simulink library "carnot"  (R2018b)
settings: Solver=VariableStepAuto  StartTime=0.0  StopTime=10.0  RelTol=1e-3
undefined symbols (not defined in the file or in its folder): A, A_earth, acol, Acol, ActPower1, ActPower2, ActPower3, Ad, Ad0, Ar, Au, Au0, Azimuth_Angle, B, Bd, Bd0, Br, Bu, Bu0, C, c1, c2, c3, c33, c4, c5, c6, CarnotCallbacks_Density, CarnotCallbacks_Enthalpy, CarnotCallbacks_Enthalpy2Temperature, CarnotCallbacks_Entropy, CarnotCallbacks_Evaporation_Enthalpy, CarnotCallbacks_GlobalMessageLevel, CarnotCallbacks_Grashof, CarnotCallbacks_Heat_Capacity, CarnotCallbacks_Kinematic_Viscosity, CarnotCallbacks_PMV_PPD, CarnotCallbacks_Prandtl, CarnotCallbacks_Saturation_Property, CarnotCallbacks_Saturation_Temperature, CarnotCallbacks_Saturation_Value_Water, CarnotCallbacks_Specific_Volume, CarnotCallbacks_Thermal_Conductivity, CarnotCallbacks_Vapour_Content, CarnotCallbacks_Vapour_Pressure, Cd, Cdl, Cr, Cu, Davies, Dd, DE_TRY2010_04_averageYear, delta_grd, density, DiameterLastPiece, dl, DPConstant, DPLinear, DPQuadratic, Dr ... (+59)
libraries: $bdroot x429, simulink x36, simulink_extras x12
(part 21 of 22)

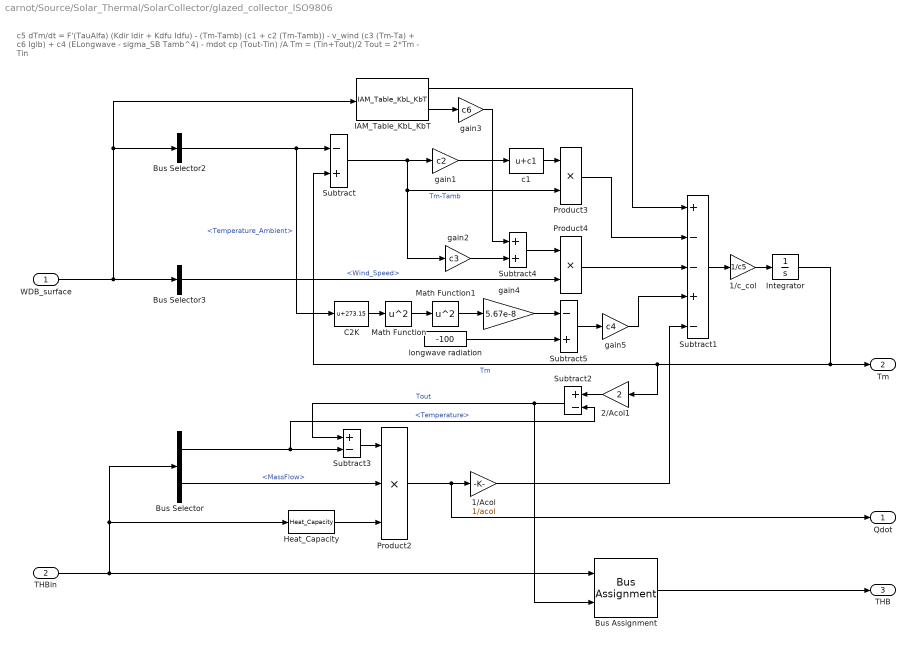
== system carnot/Source/Solar_Thermal/SolarCollector/glazed_collector_ISO9806 ==
  note: c5 dTm/dt = F'(TauAlfa) (Kdir Idir + Kdfu Idfu) - (Tm-Tamb) (c1 + c2 (Tm-Tamb)) - v_wind (c3 (Tm-Ta) + c6 Iglb) + c4 (ELongwave - sigma_SB Tamb^4) - mdot cp (Tout-Tin) /A
      | Tm = (Tin+Tout)/2
      | Tout = 2*Tm - Tin
  WDB_surface : Inport
  THBin : Inport  Port=2
  1/Acol : Gain  Gain=1/acol
  1/c_col : Gain  Gain=1/c5
  2/Acol1 : Gain  Gain=2
  Bus Assignment : BusAssignment  AssignedSignals=Temperature
  Bus Selector : BusSelector  OutputSignals=Temperature,MassFlow
  Bus Selector2 : BusSelector  OutputSignals=Temperature_Ambient
  Bus Selector3 : BusSelector  OutputSignals=Wind_Speed
  C2K : Bias  Bias=273.15
  Heat_Capacity : $bdroot/Basic/Material_Properties/Heat_Capacity  VariantControl=CarlibClassic  INPUTARGUMENTS=THB  DEBUGLEVEL=DEBUGLEVEL  MAXTOTALWARNINGS=inf  MAXCONSECUTIVEWARNINGS=inf  WRITETOFILE=0  FILENAME='errors.txt'
  IAM_Table_KbL_KbT : $bdroot/Source/Solar_Thermal/IncidenceAngleModifier/IAM_Table_KbL_KbT  fta=fta  kblangle=kblangle  KbL=KbL  kbtangle=kbtangle  KbT=KbT  Kd=Kd
  Integrator : Integrator  InitialCondition=tini
  Math Function : Math  Operator=square  SaturateOnIntegerOverflow=on
  Math Function1 : Math  Operator=square  SaturateOnIntegerOverflow=on
  Product2 : Product  Inputs=3  RndMeth=Zero
  Product3 : Product  RndMeth=Zero
  Product4 : Product  RndMeth=Zero
  Subtract : Sum  Inputs=-+
  Subtract1 : Sum  Inputs=+--+-
  Subtract2 : Sum  Inputs=+-
  Subtract3 : Sum  Inputs=+-
  Subtract4 : Sum  Inputs=2
  Subtract5 : Sum  Inputs=-+
  c1 : Bias  Bias=c1
  gain1 : Gain  Gain=c2
  gain2 : Gain  Gain=c3
  gain3 : Gain  Gain=c6
  gain4 : Gain  Gain=5.67e-8
  gain5 : Gain  Gain=c4
  longwave radiation : Constant  Value=-100
  Qdot : Outport  InitialOutput=0
  Tm : Outport  Port=2  InitialOutput=0
  THB : Outport  Port=3  InitialOutput=0
  wires:
  WDB_surface/1 -> Bus Selector3/1, IAM_Table_KbL_KbT/1, Bus Selector2/1
  Subtract4/1 -> Product4/1
  C2K/1 -> Math Function/1
  longwave radiation/1 -> Subtract5/2
  gain5/1 -> Subtract1/4
  Math Function/1 -> Math Function1/1
  2/Acol1/1 -> Subtract2/1
  Subtract/1 -> gain1/1, Product3/2, gain2/1  "Tm-Tamb"
  1/Acol/1 -> Subtract1/5
  Subtract2/1 -> Bus Assignment/2, Subtract3/1  "Tout"
  Heat_Capacity/1 -> Product2/3
  Integrator/1 -> Tm/1, 2/Acol1/1, Subtract/2  "Tm"
  Product2/1 -> Qdot/1, 1/Acol/1
  IAM_Table_KbL_KbT/2 -> gain3/1
  Subtract3/1 -> Product2/1
  Bus Selector2/1 -> C2K/1, Subtract/1  "<Temperature_Ambient>"
  gain1/1 -> c1/1
  gain2/1 -> Subtract4/2
  Product3/1 -> Subtract1/2
  1/c_col/1 -> Integrator/1
  Product4/1 -> Subtract1/3
  Math Function1/1 -> gain4/1
  THBin/1 -> Bus Assignment/1, Heat_Capacity/1, Bus Selector/1
  IAM_Table_KbL_KbT/1 -> Subtract1/1
  Bus Selector3/1 -> Product4/2  "<Wind_Speed>"
  Subtract5/1 -> gain5/1
  gain3/1 -> Subtract4/1
  gain4/1 -> Subtract5/1
  Subtract1/1 -> 1/c_col/1
  c1/1 -> Product3/1
  Bus Selector/1 -> Subtract2/2, Subtract3/2  "<Temperature>"
  Bus Selector/2 -> Product2/2  "<MassFlow>"
  Bus Assignment/1 -> THB/1

== system carnot/Source/Solar_Thermal/SolarCollector_2node/create_Cdat ==
  acol : Inport
  THBin : Inport  Port=2
  THBout : Inport  Port=3
  Qdot : Inport  Port=4
  Tmean : Inport  Port=5
  WDB : Inport  Port=6
  Bus Creator : BusCreator  Inputs=6
  Cdat : Outport
  wires:
  acol/1 -> Bus Creator/1  "Acol"
  THBin/1 -> Bus Creator/2  "THBin"
  THBout/1 -> Bus Creator/3  "THBout"
  WDB/1 -> Bus Creator/6  "WDB_surface"
  Bus Creator/1 -> Cdat/1
  Qdot/1 -> Bus Creator/4  "Qdot"
  Tmean/1 -> Bus Creator/5  "Tmean"

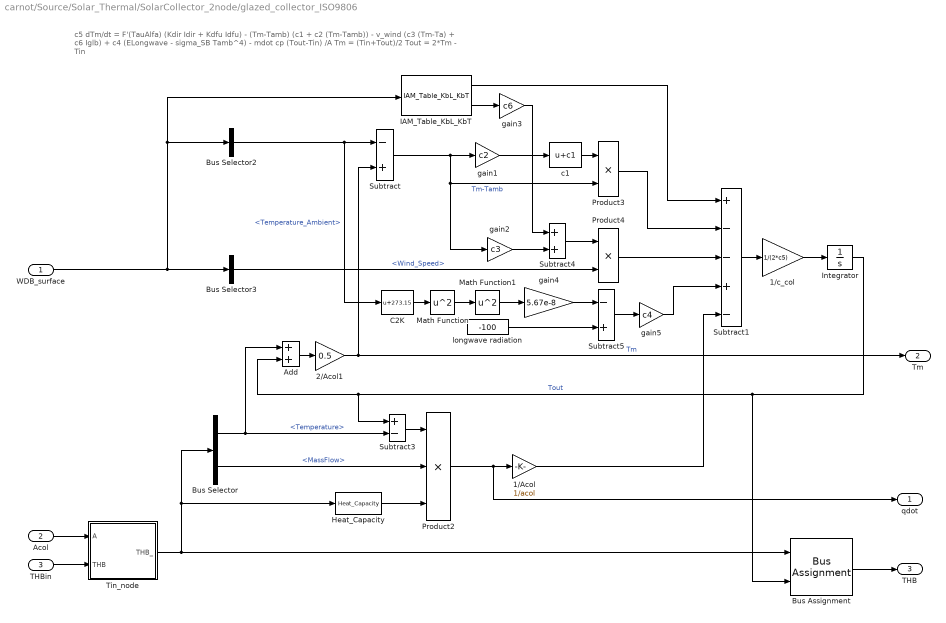
== system carnot/Source/Solar_Thermal/SolarCollector_2node/glazed_collector_ISO9806 ==
  note: c5 dTm/dt = F'(TauAlfa) (Kdir Idir + Kdfu Idfu) - (Tm-Tamb) (c1 + c2 (Tm-Tamb)) - v_wind (c3 (Tm-Ta) + c6 Iglb) + c4 (ELongwave - sigma_SB Tamb^4) - mdot cp (Tout-Tin) /A
      | Tm = (Tin+Tout)/2
      | Tout = 2*Tm - Tin
  WDB_surface : Inport
  Acol : Inport  Port=2
  THBin : Inport  Port=3
  1/Acol : Gain  Gain=1/acol
  1/c_col : Gain  Gain=1/(2*c5)
  2/Acol1 : Gain  Gain=0.5
  Add : Sum
  Bus Assignment : BusAssignment  AssignedSignals=Temperature
  Bus Selector : BusSelector  OutputSignals=Temperature,MassFlow
  Bus Selector2 : BusSelector  OutputSignals=Temperature_Ambient
  Bus Selector3 : BusSelector  OutputSignals=Wind_Speed
  C2K : Bias  Bias=273.15
  Heat_Capacity : $bdroot/Basic/Material_Properties/Heat_Capacity  VariantControl=CarlibClassic  INPUTARGUMENTS=THB  DEBUGLEVEL=DEBUGLEVEL  MAXTOTALWARNINGS=inf  MAXCONSECUTIVEWARNINGS=inf  WRITETOFILE=0  FILENAME='errors.txt'
  IAM_Table_KbL_KbT : $bdroot/Source/Solar_Thermal/IncidenceAngleModifier/IAM_Table_KbL_KbT  fta=fta  kblangle=kblangle  KbL=KbL  kbtangle=kbtangle  KbT=KbT  Kd=Kd
  Integrator : Integrator  InitialCondition=tini
  Math Function : Math  Operator=square  SaturateOnIntegerOverflow=on
  Math Function1 : Math  Operator=square  SaturateOnIntegerOverflow=on
  Product2 : Product  Inputs=3  RndMeth=Zero
  Product3 : Product  RndMeth=Zero
  Product4 : Product  RndMeth=Zero
  Subtract : Sum  Inputs=-+
  Subtract1 : Sum  Inputs=+--+-
  Subtract3 : Sum  Inputs=+-
  Subtract4 : Sum  Inputs=2
  Subtract5 : Sum  Inputs=-+
  Tin_node : Subsystem
  c1 : Bias  Bias=c1
  gain1 : Gain  Gain=c2
  gain2 : Gain  Gain=c3
  gain3 : Gain  Gain=c6
  gain4 : Gain  Gain=5.67e-8
  gain5 : Gain  Gain=c4
  longwave radiation : Constant  Value=-100
  qdot : Outport  InitialOutput=0
  Tm : Outport  Port=2  InitialOutput=0
  THB : Outport  Port=3  InitialOutput=0
  wires:
  Add/1 -> 2/Acol1/1
  2/Acol1/1 -> Subtract/2, Tm/1  "Tm"
  Acol/1 -> Tin_node/1(A)
  THBin/1 -> Tin_node/2(THB)
  WDB_surface/1 -> Bus Selector3/1, IAM_Table_KbL_KbT/1, Bus Selector2/1
  Subtract4/1 -> Product4/1
  C2K/1 -> Math Function/1
  longwave radiation/1 -> Subtract5/2
  gain5/1 -> Subtract1/4
  Math Function/1 -> Math Function1/1
  Subtract/1 -> gain1/1, Product3/2, gain2/1  "Tm-Tamb"
  1/Acol/1 -> Subtract1/5
  Heat_Capacity/1 -> Product2/3
  Integrator/1 -> Bus Assignment/2, Add/2, Subtract3/1  "Tout"
  Product2/1 -> qdot/1, 1/Acol/1
  IAM_Table_KbL_KbT/2 -> gain3/1
  Subtract3/1 -> Product2/1
  Bus Selector2/1 -> C2K/1, Subtract/1  "<Temperature_Ambient>"
  gain1/1 -> c1/1
  gain2/1 -> Subtract4/2
  Product3/1 -> Subtract1/2
  1/c_col/1 -> Integrator/1
  Product4/1 -> Subtract1/3
  Math Function1/1 -> gain4/1
  Tin_node/1(THB_) -> Heat_Capacity/1, Bus Selector/1, Bus Assignment/1
  IAM_Table_KbL_KbT/1 -> Subtract1/1
  Bus Selector3/1 -> Product4/2  "<Wind_Speed>"
  Subtract5/1 -> gain5/1
  gain3/1 -> Subtract4/1
  gain4/1 -> Subtract5/1
  Subtract1/1 -> 1/c_col/1
  c1/1 -> Product3/1
  Bus Selector/1 -> Add/1, Subtract3/2  "<Temperature>"
  Bus Selector/2 -> Product2/2  "<MassFlow>"
  Bus Assignment/1 -> THB/1

== system carnot/Source/Ventilation/Ventilation_AIV/Subsystem ==
  note: Remaining humidity or CO2 concentration
      | is difference of incomming x from outside (x_out)
      | and leaving x from inside (x_in)
  note: (kg/s)
  note: (kg/s)
  note: (kg/s)
  note: (kg/kg)
  note: (kg/kg)
  note: ASSUMPTION: mdot_air_out2in is equal to mdot_air_in2out
      | for the entire building
  mdot_air : Inport
  x_in : Inport  Port=2
  x_out : Inport  Port=3
  Constant : Constant  Value=0
  Demux2 : Demux  Outputs=2
  Demux3 : Demux  Outputs=2
  Product5 : Product  SaturateOnIntegerOverflow=on  InputSameDT=on  OutDataTypeStr=Inherit: Same as first input
  Product6 : Product  SaturateOnIntegerOverflow=on  InputSameDT=on  OutDataTypeStr=Inherit: Same as first input
  Sum1 : Sum  Inputs=+-  SaturateOnIntegerOverflow=on  InputSameDT=on  OutDataTypeStr=Inherit: Same as first input
  Sum2 : Sum  Inputs=+-  SaturateOnIntegerOverflow=on  InputSameDT=on  OutDataTypeStr=Inherit: Same as first input
  D_mdot_air : Outport
  D_mdot_H2O : Outport  Port=2
  D_mdot_CO2 : Outport  Port=3
  wires:
  x_out/1 -> Demux2/1
  Demux2/1 -> Sum1/1  "x_H2O_out"
  Demux2/2 -> Sum2/1  "x_CO2_out"
  Demux3/2 -> Sum2/2  "x_CO2_in"
  Demux3/1 -> Sum1/2  "x_H2O_in"
  x_in/1 -> Demux3/1
  Sum2/1 -> Product6/2
  Sum1/1 -> Product5/2
  mdot_air/1 -> Product5/1, Product6/1  "mdot_air"
  Product6/1 -> D_mdot_CO2/1  "mdot_CO2"
  Product5/1 -> D_mdot_H2O/1  "mdot_H2O"
  Constant/1 -> D_mdot_air/1

== system carnot/Storage/Thermal/Ice_Storage/Heat_Exchanger_HP ==
  note: 1.5 kW at 9 K on a 28 m tube
  Tice : Inport
  Tin : Inport  Port=2
  mdot : Inport  Port=3
  p : Inport  Port=4
  fluid : Inport  Port=5
  mix : Inport  Port=6
  Constant : Constant  Value=Lhx
  Constant1 : Constant  Value=mpc_hp
  Heat_Capacity : $bdroot/Basic/Material_Properties/Heat_Capacity  VariantControl=CarlibClassic  INPUTARGUMENTS=state variables (classic)  DEBUGLEVEL=DEBUGLEVEL  MAXTOTALWARNINGS=inf  MAXCONSECUTIVEWARNINGS=inf  WRITETOFILE=0  FILENAME='errors.txt'
  Integrator : Integrator  InitialCondition=t_ini
  Multiply : Product
  Multiply1 : Product  Inputs=/*/
  Product : Product  Inputs=3  SaturateOnIntegerOverflow=on  InputSameDT=on  OutDataTypeStr=Inherit: Same as first input
  Sum : Sum  Inputs=-+  SaturateOnIntegerOverflow=on  InputSameDT=on  OutDataTypeStr=Inherit: Same as first input
  Sum1 : Sum  Inputs=-+  SaturateOnIntegerOverflow=on  InputSameDT=on  OutDataTypeStr=Inherit: Same as first input
  Sum2 : Sum  Inputs=+-  SaturateOnIntegerOverflow=on  InputSameDT=on  OutDataTypeStr=Inherit: Same as first input
  U_length : Gain  Gain=Ulen  SaturateOnIntegerOverflow=on  OutDataTypeStr=Inherit: Same as input  ParamDataTypeStr=Inherit: Same as input
  Qdot2ice : Outport
  Thx : Outport  Port=2
  wires:
  Sum1/1 -> Multiply1/2
  Multiply1/1 -> Integrator/1
  Constant1/1 -> Multiply1/3
  Constant/1 -> Multiply/1, Multiply1/1
  Multiply/1 -> Sum1/1, Qdot2ice/1
  U_length/1 -> Multiply/2
  Tice/1 -> Sum2/2
  mix/1 -> Heat_Capacity/4
  fluid/1 -> Heat_Capacity/3
  p/1 -> Heat_Capacity/2
  mdot/1 -> Product/2
  Sum2/1 -> U_length/1
  Sum/1 -> Product/1
  Heat_Capacity/1 -> Product/3
  Product/1 -> Sum1/2
  Integrator/1 -> Thx/1, Sum2/1, Sum/1  "Thx"
  Tin/1 -> Sum/2, Heat_Capacity/1

== system carnot/Storage/Thermal/Ice_Storage/Heat_Exchanger_Solar ==
  note: 1.5 kW at 9 K on a 28 m tube
  Tice : Inport
  Tin : Inport  Port=2
  mdot : Inport  Port=3
  p : Inport  Port=4
  fluid : Inport  Port=5
  mix : Inport  Port=6
  Constant : Constant  Value=Lhx
  Constant1 : Constant  Value=mpc_hp
  Heat_Capacity : $bdroot/Basic/Material_Properties/Heat_Capacity  VariantControl=CarlibClassic  INPUTARGUMENTS=state variables (classic)  DEBUGLEVEL=DEBUGLEVEL  MAXTOTALWARNINGS=inf  MAXCONSECUTIVEWARNINGS=inf  WRITETOFILE=0  FILENAME='errors.txt'
  Integrator : Integrator  InitialCondition=t_ini
  Multiply : Product
  Multiply1 : Product  Inputs=/*/
  Product : Product  Inputs=3  SaturateOnIntegerOverflow=on  InputSameDT=on  OutDataTypeStr=Inherit: Same as first input
  Sum : Sum  Inputs=-+  SaturateOnIntegerOverflow=on  InputSameDT=on  OutDataTypeStr=Inherit: Same as first input
  Sum1 : Sum  Inputs=-+  SaturateOnIntegerOverflow=on  InputSameDT=on  OutDataTypeStr=Inherit: Same as first input
  Sum2 : Sum  Inputs=+-  SaturateOnIntegerOverflow=on  InputSameDT=on  OutDataTypeStr=Inherit: Same as first input
  U_length : Gain  Gain=Ulen  SaturateOnIntegerOverflow=on  OutDataTypeStr=Inherit: Same as input  ParamDataTypeStr=Inherit: Same as input
  Qdot2ice : Outport
  Thx : Outport  Port=2
  wires:
  Tin/1 -> Heat_Capacity/1, Sum/2
  Integrator/1 -> Sum/1, Sum2/1, Thx/1  "Thx"
  Product/1 -> Sum1/2
  Heat_Capacity/1 -> Product/3
  Sum/1 -> Product/1
  Sum2/1 -> U_length/1
  mdot/1 -> Product/2
  p/1 -> Heat_Capacity/2
  fluid/1 -> Heat_Capacity/3
  mix/1 -> Heat_Capacity/4
  Tice/1 -> Sum2/2
  U_length/1 -> Multiply/2
  Multiply/1 -> Qdot2ice/1, Sum1/1
  Constant/1 -> Multiply1/1, Multiply/1
  Constant1/1 -> Multiply1/3
  Multiply1/1 -> Integrator/1
  Sum1/1 -> Multiply1/2

== system carnot/Storage/Thermal/Ice_Storage/T_ground_undisturbed ==
  Fcn : Fcn  Expr=u(1) - u(2)*exp(-u(3)/u(4))*cos(2*pi*(u(5)-u(6)*3600)/(365*24*3600) - u(3)/u(4)) + 0.03*u(3)
  Mux : Mux  Inputs=6
  Tmeanoutside : Constant  Value=Tmeanoutside
  delta_grd : Constant  Value=delta_grd
  deltathetae : Constant  Value=deltathetae
  depth of center of wall : Constant  Value=ztilde
  time : Clock
  tshift : Constant  Value=tshift
  Tearth : Outport
  wires:
  Tmeanoutside/1 -> Mux/1
  deltathetae/1 -> Mux/2
  depth of center of wall/1 -> Mux/3
  delta_grd/1 -> Mux/4
  time/1 -> Mux/5
  tshift/1 -> Mux/6
  Mux/1 -> Fcn/1
  Fcn/1 -> Tearth/1

== system carnot/Storage/Thermal/Storage_Ports/Electric_Heating ==
  electric power : Inport
  THB : Inport  Port=2
  Bus Selector : BusSelector  OutputSignals=FluidType,FluidMix
  Gain : Gain  Gain=Q
  Mux3 : Mux  Inputs=8
  T_in : Constant  Value=ones(nodes,1)*20
  const2 : Constant  Value=1e5
  mdot : Constant  Value=zeros(nodes,1)
  to_storeT : Outport
  wires:
  Gain/1 -> Mux3/5  "Qdot_in"
  Bus Selector/2 -> Mux3/8  "<FluidMix>"
  electric power/1 -> Gain/1
  T_in/1 -> Mux3/1  "T_in"
  Mux3/1 -> to_storeT/1
  mdot/1 -> Mux3/4, Mux3/3, Mux3/2  "mdot_in"
  const2/1 -> Mux3/6
  THB/1 -> Bus Selector/1
  Bus Selector/1 -> Mux3/7  "<FluidType>"

== system carnot/Storage/Thermal/Storage_Ports/HX_EN12977 ==
  from_storeT : Inport
  THBin : Inport  Port=2
  Bus Assignment1 : BusAssignment  AssignedSignals=Temperature
  Mux3 : Mux  Inputs=8
  Pressure_Drop_StorageHX : $bdroot/Basic/Pressure_Drop/Pressure_Drop_StorageHX  dia=dia  hgt=height  dplin=dplin  dpqua=dpqua
  T_in : Constant  Value=zeros(nodes,1)
  fluid : Constant  Value=-9999
  mdot_in : Constant  Value=zeros(nodes,1)
  mix : Constant  Value=-9999
  p : Constant  Value=-9999
  select_Tout : Selector  InputPortWidth=nodes  IndexOptions=Index vector (dialog)  Indices=[outlet]  OutputSizes=1
  sfun_storage_heatexchanger : $bdroot/Basic/Thermal_Models/sfun_storage_heatexchanger  idn=heat transfer data fit EN12977  nodes=nodes  inlet=inlet  outlet=outlet  p1=ua0  p2=uam  p3=uat  p4=uat2  p5=0  p6=0  p7=0
  to_storeT : Outport
  THBout : Outport  Port=2
  wires:
  from_storeT/1 -> sfun_storage_heatexchanger/1
  THBin/1 -> Pressure_Drop_StorageHX/1, sfun_storage_heatexchanger/2
  mdot_in/1 -> Mux3/2, Mux3/3, Mux3/4  "mdot_in"
  Mux3/1 -> to_storeT/1
  select_Tout/1 -> Bus Assignment1/2
  T_in/1 -> Mux3/1  "T_in"
  sfun_storage_heatexchanger/1 -> Mux3/5  "Q_in"
  Bus Assignment1/1 -> THBout/1
  p/1 -> Mux3/6
  fluid/1 -> Mux3/7
  mix/1 -> Mux3/8
  sfun_storage_heatexchanger/2 -> select_Tout/1
  Pressure_Drop_StorageHX/1 -> Bus Assignment1/1

== system carnot/Storage/Thermal/Storage_Ports/HX_EN12977_stratified ==
  from_storeT : Inport
  THBin : Inport  Port=2
  Bus Assignment1 : BusAssignment  AssignedSignals=Temperature
  Mux3 : Mux  Inputs=8
  Pressure_Drop_StorageHX : $bdroot/Basic/Pressure_Drop/Pressure_Drop_StorageHX  dia=dia  hgt=height  dplin=dplin  dpqua=dpqua
  T_in : Constant  Value=zeros(nodes,1)
  fluid : Constant  Value=-9999
  mdot_in : Constant  Value=zeros(nodes,1)
  mix : Constant  Value=-9999
  p : Constant  Value=-9999
  select_Tout : Selector  InputPortWidth=nodes  IndexOptions=Index vector (dialog)  Indices=[outlet]  OutputSizes=1
  sfun_storage_heatexchanger : $bdroot/Basic/Thermal_Models/sfun_storage_heatexchanger  idn="heat transfer data fit EN12977  - stratified"  nodes=nodes  inlet=inlet  outlet=outlet  p1=ua0  p2=uam  p3=uat  p4=uat2  p5=0  p6=0  p7=0
  to_storeT : Outport
  THBout : Outport  Port=2
  wires:
  from_storeT/1 -> sfun_storage_heatexchanger/1
  THBin/1 -> Pressure_Drop_StorageHX/1, sfun_storage_heatexchanger/2
  mdot_in/1 -> Mux3/2, Mux3/3, Mux3/4  "mdot_in"
  Mux3/1 -> to_storeT/1
  select_Tout/1 -> Bus Assignment1/2
  T_in/1 -> Mux3/1  "T_in"
  sfun_storage_heatexchanger/1 -> Mux3/5  "Q_in"
  Bus Assignment1/1 -> THBout/1
  p/1 -> Mux3/6
  fluid/1 -> Mux3/7
  mix/1 -> Mux3/8
  sfun_storage_heatexchanger/2 -> select_Tout/1
  Pressure_Drop_StorageHX/1 -> Bus Assignment1/1

== system carnot/Storage/Thermal/Storage_Ports/HX_data_fit ==
  note: UA = uac + mdot*uam + (Thx-Tstorage)*uat
      | Qdot = UA * (Tstore-Thx)
  from_storeT : Inport
  THBin : Inport  Port=2
  Bus Assignment1 : BusAssignment  AssignedSignals=Temperature
  Mux3 : Mux  Inputs=8
  Pressure_Drop_StorageHX : $bdroot/Basic/Pressure_Drop/Pressure_Drop_StorageHX  dia=dia  hgt=height  dplin=dplin  dpqua=dpqua
  T_in : Constant  Value=zeros(nodes,1)
  fluid : Constant  Value=-9999
  mdot_in : Constant  Value=zeros(nodes,1)
  mix : Constant  Value=-9999
  p : Constant  Value=-9999
  select_Tout : Selector  InputPortWidth=nodes  IndexOptions=Index vector (dialog)  Indices=[outlet]  OutputSizes=1
  sfun_storage_heatexchanger : $bdroot/Basic/Thermal_Models/sfun_storage_heatexchanger  idn=heat transfer from data fit  nodes=nodes  inlet=inlet  outlet=outlet  p1=ua0  p2=uam  p3=uat  p4=0  p5=0  p6=0  p7=0
  to_storeT : Outport
  THBout : Outport  Port=2
  wires:
  sfun_storage_heatexchanger/2 -> select_Tout/1
  mix/1 -> Mux3/8
  fluid/1 -> Mux3/7
  p/1 -> Mux3/6
  Bus Assignment1/1 -> THBout/1
  sfun_storage_heatexchanger/1 -> Mux3/5  "Q_in"
  T_in/1 -> Mux3/1  "T_in"
  select_Tout/1 -> Bus Assignment1/2
  Mux3/1 -> to_storeT/1
  mdot_in/1 -> Mux3/4, Mux3/3, Mux3/2  "mdot_in"
  THBin/1 -> Pressure_Drop_StorageHX/1, sfun_storage_heatexchanger/2
  from_storeT/1 -> sfun_storage_heatexchanger/1
  Pressure_Drop_StorageHX/1 -> Bus Assignment1/1

== system carnot/Storage/Thermal/Storage_Ports/HX_data_fit_stratified ==
  note: statified charging !
      | heat transfer:
      | UA = uac + mdot*uam + (Thx-Tstorage)*uat
      | Qdot = UA * (Tstore-Thx)
  from_storeT : Inport
  THBin : Inport  Port=2
  Bus Assignment1 : BusAssignment  AssignedSignals=Temperature
  Mux3 : Mux  Inputs=8
  Pressure_Drop_StorageHX : $bdroot/Basic/Pressure_Drop/Pressure_Drop_StorageHX  dia=dia  hgt=height  dplin=dplin  dpqua=dpqua
  T_in : Constant  Value=zeros(nodes,1)
  fluid : Constant  Value=-9999
  mdot_in : Constant  Value=zeros(nodes,1)
  mix : Constant  Value=-9999
  p : Constant  Value=-9999
  select_Tout : Selector  InputPortWidth=nodes  IndexOptions=Index vector (dialog)  Indices=[outlet]  OutputSizes=1
  sfun_storage_heatexchanger : $bdroot/Basic/Thermal_Models/sfun_storage_heatexchanger  idn="heat transfer from data fit  - stratified"  nodes=nodes  inlet=inlet  outlet=outlet  p1=ua0  p2=uam  p3=uat  p4=0  p5=0  p6=0  p7=0
  to_storeT : Outport
  THBout : Outport  Port=2
  wires:
  from_storeT/1 -> sfun_storage_heatexchanger/1
  THBin/1 -> Pressure_Drop_StorageHX/1, sfun_storage_heatexchanger/2
  mdot_in/1 -> Mux3/2, Mux3/3, Mux3/4  "mdot_in"
  Mux3/1 -> to_storeT/1
  select_Tout/1 -> Bus Assignment1/2
  T_in/1 -> Mux3/1  "T_in"
  sfun_storage_heatexchanger/1 -> Mux3/5  "Q_in"
  p/1 -> Mux3/6
  fluid/1 -> Mux3/7
  mix/1 -> Mux3/8
  sfun_storage_heatexchanger/2 -> select_Tout/1
  Pressure_Drop_StorageHX/1 -> Bus Assignment1/1
  Bus Assignment1/1 -> THBout/1

== system carnot/Storage/Thermal/Storage_Ports/HX_finned_tube ==
  from_storeT : Inport
  THBin : Inport  Port=2
  Bus Assignment1 : BusAssignment  AssignedSignals=Temperature
  Mux3 : Mux  Inputs=8
  Pressure_Drop_StorageHX : $bdroot/Basic/Pressure_Drop/Pressure_Drop_StorageHX  dia=dpipe  hgt=height  dplin=dplin  dpqua=dpqua
  T_in : Constant  Value=zeros(nodes,1)
  fluid : Constant  Value=-9999
  mdot_in : Constant  Value=zeros(nodes,1)
  mix : Constant  Value=-9999
  p : Constant  Value=-9999
  select_Tout : Selector  InputPortWidth=nodes  IndexOptions=Index vector (dialog)  Indices=[outlet]  OutputSizes=1
  sfun_storage_heatexchanger : $bdroot/Basic/Thermal_Models/sfun_storage_heatexchanger  idn=finned tube theoretical  nodes=nodes  inlet=inlet  outlet=outlet  p1=dpipe  p2=swall  p3=lpipe  p4=cond  p5=dfin  p6=sfin  p7=nfin
  to_storeT : Outport
  THBout : Outport  Port=2
  wires:
  from_storeT/1 -> sfun_storage_heatexchanger/1
  THBin/1 -> Pressure_Drop_StorageHX/1, sfun_storage_heatexchanger/2
  mdot_in/1 -> Mux3/2, Mux3/3, Mux3/4  "mdot_in"
  Mux3/1 -> to_storeT/1
  select_Tout/1 -> Bus Assignment1/2
  T_in/1 -> Mux3/1  "T_in"
  sfun_storage_heatexchanger/1 -> Mux3/5  "Q_in"
  Bus Assignment1/1 -> THBout/1
  p/1 -> Mux3/6
  fluid/1 -> Mux3/7
  mix/1 -> Mux3/8
  sfun_storage_heatexchanger/2 -> select_Tout/1
  Pressure_Drop_StorageHX/1 -> Bus Assignment1/1

== system carnot/Storage/Thermal/Storage_Ports/HX_finned_tube_stratified ==
  from_storeT : Inport
  THBin : Inport  Port=2
  Bus Assignment1 : BusAssignment  AssignedSignals=Temperature
  Mux3 : Mux  Inputs=8
  Pressure_Drop_StorageHX : $bdroot/Basic/Pressure_Drop/Pressure_Drop_StorageHX  dia=dpipe  hgt=height  dplin=dplin  dpqua=dpqua
  T_in : Constant  Value=zeros(nodes,1)
  fluid : Constant  Value=-9999
  mdot_in : Constant  Value=zeros(nodes,1)
  mix : Constant  Value=-9999
  p : Constant  Value=-9999
  select_Tout : Selector  InputPortWidth=nodes  IndexOptions=Index vector (dialog)  Indices=[outlet]  OutputSizes=1
  sfun_storage_heatexchanger : $bdroot/Basic/Thermal_Models/sfun_storage_heatexchanger  idn="finned tube theoretical  - stratified"  nodes=nodes  inlet=inlet  outlet=outlet  p1=dpipe  p2=swall  p3=lpipe  p4=cond  p5=dfin  p6=sfin  p7=nfin
  to_storeT : Outport
  THBout : Outport  Port=2
  wires:
  Pressure_Drop_StorageHX/1 -> Bus Assignment1/1
  sfun_storage_heatexchanger/2 -> select_Tout/1
  mix/1 -> Mux3/8
  fluid/1 -> Mux3/7
  p/1 -> Mux3/6
  Bus Assignment1/1 -> THBout/1
  sfun_storage_heatexchanger/1 -> Mux3/5  "Q_in"
  T_in/1 -> Mux3/1  "T_in"
  select_Tout/1 -> Bus Assignment1/2
  Mux3/1 -> to_storeT/1
  mdot_in/1 -> Mux3/4, Mux3/3, Mux3/2  "mdot_in"
  THBin/1 -> sfun_storage_heatexchanger/2, Pressure_Drop_StorageHX/1
  from_storeT/1 -> sfun_storage_heatexchanger/1

== system carnot/Storage/Thermal/Storage_Ports/HX_tube ==
  from_storeT : Inport
  THBin : Inport  Port=2
  Bus Assignment1 : BusAssignment  AssignedSignals=Temperature
  Mux3 : Mux  Inputs=8
  Pressure_Drop_StorageHX : $bdroot/Basic/Pressure_Drop/Pressure_Drop_StorageHX  dia=dia  hgt=height  dplin=dplin  dpqua=dpqua
  T_in : Constant  Value=zeros(nodes,1)
  fluid : Constant  Value=-9999
  mdot_in : Constant  Value=zeros(nodes,1)
  mix : Constant  Value=-9999
  p : Constant  Value=-9999
  select_Tout : Selector  InputPortWidth=nodes  IndexOptions=Index vector (dialog)  Indices=[outlet]  OutputSizes=1
  sfun_storage_heatexchanger : $bdroot/Basic/Thermal_Models/sfun_storage_heatexchanger  idn=smooth tube theoretical  nodes=nodes  inlet=inlet  outlet=outlet  p1=dpipe  p2=swall  p3=lpipe  p4=cond  p5=0  p6=0  p7=0
  to_storeT : Outport
  THBout : Outport  Port=2
  wires:
  Pressure_Drop_StorageHX/1 -> Bus Assignment1/1
  sfun_storage_heatexchanger/2 -> select_Tout/1
  mix/1 -> Mux3/8
  fluid/1 -> Mux3/7
  p/1 -> Mux3/6
  Bus Assignment1/1 -> THBout/1
  sfun_storage_heatexchanger/1 -> Mux3/5  "Q_in"
  T_in/1 -> Mux3/1  "T_in"
  select_Tout/1 -> Bus Assignment1/2
  Mux3/1 -> to_storeT/1
  mdot_in/1 -> Mux3/4, Mux3/3, Mux3/2  "mdot_in"
  THBin/1 -> Pressure_Drop_StorageHX/1, sfun_storage_heatexchanger/2
  from_storeT/1 -> sfun_storage_heatexchanger/1

== system carnot/Storage/Thermal/Storage_Ports/HX_tube_stratified ==
  from_storeT : Inport
  THBin : Inport  Port=2
  Bus Assignment1 : BusAssignment  AssignedSignals=Temperature
  Mux3 : Mux  Inputs=8
  Pressure_Drop_StorageHX : $bdroot/Basic/Pressure_Drop/Pressure_Drop_StorageHX  dia=dia  hgt=height  dplin=dplin  dpqua=dpqua
  T_in : Constant  Value=zeros(nodes,1)
  fluid : Constant  Value=-9999
  mdot_in : Constant  Value=zeros(nodes,1)
  mix : Constant  Value=-9999
  p : Constant  Value=-9999
  select_Tout : Selector  InputPortWidth=nodes  IndexOptions=Index vector (dialog)  Indices=[outlet]  OutputSizes=1
  sfun_storage_heatexchanger : $bdroot/Basic/Thermal_Models/sfun_storage_heatexchanger  idn=smooth tube theoretical - stratified  nodes=nodes  inlet=inlet  outlet=outlet  p1=dpipe  p2=swall  p3=lpipe  p4=cond  p5=0  p6=0  p7=0
  to_storeT : Outport
  THBout : Outport  Port=2
  wires:
  from_storeT/1 -> sfun_storage_heatexchanger/1
  THBin/1 -> sfun_storage_heatexchanger/2, Pressure_Drop_StorageHX/1
  mdot_in/1 -> Mux3/2, Mux3/3, Mux3/4  "mdot_in"
  Mux3/1 -> to_storeT/1
  select_Tout/1 -> Bus Assignment1/2
  T_in/1 -> Mux3/1  "T_in"
  sfun_storage_heatexchanger/1 -> Mux3/5  "Q_in"
  Bus Assignment1/1 -> THBout/1
  p/1 -> Mux3/6
  fluid/1 -> Mux3/7
  mix/1 -> Mux3/8
  sfun_storage_heatexchanger/2 -> select_Tout/1
  Pressure_Drop_StorageHX/1 -> Bus Assignment1/1

== system carnot/Storage/Thermal/Storage_Ports/Pipe_Connection ==
  from_storeT : Inport
  THBin : Inport  Port=2
  Bus Assignment : BusAssignment  AssignedSignals=Temperature
  Bus Selector : BusSelector  OutputSignals=Temperature,MassFlow,Pressure,FluidType,FluidMix
  Gain : Gain  Gain=in
  Gain1 : Gain  Gain=up
  Gain2 : Gain  Gain=down
  Gain3 : Gain  Gain=in
  Mux3 : Mux  Inputs=8
  Pressure_Drop_StoragePipe : $bdroot/Basic/Pressure_Drop/Pressure_Drop_StoragePipe  dpipe=dpipe  dstg=dstg  hgt=height
  Q_in : Constant  Value=zeros(nodes,1)
  select_Tin_2_Tout : Selector  InputPortWidth=nodes  IndexOptions=Index vector (dialog)  Indices=[idx_in_out]  OutputSizes=1
  select_Tout : Selector  InputPortWidth=nodes  IndexOptions=Index vector (dialog)  Indices=[outlet]  OutputSizes=1
  to_storeT : Outport
  THBout : Outport  Port=2
  wires:
  select_Tin_2_Tout/1 -> Pressure_Drop_StoragePipe/1
  Bus Selector/5 -> Mux3/8  "<FluidMix>"
  Bus Assignment/1 -> THBout/1
  Q_in/1 -> Mux3/5
  Gain3/1 -> Mux3/1  "T_in"
  select_Tout/1 -> Bus Assignment/2
  Mux3/1 -> to_storeT/1
  Gain2/1 -> Mux3/4  "mdot_down"
  Gain1/1 -> Mux3/3  "mdot_up"
  Gain/1 -> Mux3/2  "mdot_in"
  Bus Selector/1 -> Gain3/1  "<Temperature>"
  Bus Selector/2 -> Gain2/1, Gain1/1, Gain/1  "<MassFlow>"
  Bus Selector/3 -> Mux3/6  "<Pressure>"
  Bus Selector/4 -> Mux3/7  "<FluidType>"
  THBin/1 -> Bus Selector/1, Pressure_Drop_StoragePipe/2
  from_storeT/1 -> select_Tin_2_Tout/1, select_Tout/1
  Pressure_Drop_StoragePipe/1 -> Bus Assignment/1

== system carnot/Storage/Thermal/Storage_Ports/Pipe_stratified ==
  note: _________________________________
      | mdot_in ->                                                .
      | node 5                     .
      | __ mdot_down(4) V  ___mdot_up(4) ^ __
      | V                           ^    .
      | node 4                    .
      | __ mdot_down(3) V  ___mdot_up(3) ^ __
      | V                           ^    .
      | node 3                    .
      | __ mdot_down(2) V  ___mdot_up(2) ^ __
      | V                           ^    .
      | node 2                    .
      | __ mdot_down(1) V  ___mdot_up(1) ^ __
      | V                           ^    .
      | node 1                    .
      | _________________________________
  from_storeT : Inport
  THBin : Inport  Port=2
  Add : Sum  Inputs=-+
  Add2 : Sum  Inputs=1
  Bus Assignment : BusAssignment  AssignedSignals=Temperature
  Bus Selector : BusSelector  OutputSignals=Temperature,MassFlow,Pressure,FluidType,FluidMix
  Constant : Constant  Value=flowdir
  Gain1 : Gain  Gain=up
  Gain2 : Gain  Gain=flowdir
  Gain3 : Gain  Gain=ones(nodes,1)
  Gain5 : Gain  Gain=down
  If : If  NumInputs=2  IfExpression=u1 == 0  ElseIfExpressions=u2 < 0
  MinMax : MinMax  Function=max  Inputs=3
  Mux3 : Mux  Inputs=8
  Pressure_Drop_StoragePipe : $bdroot/Basic/Pressure_Drop/Pressure_Drop_StoragePipe  dpipe=dpipe  dstg=dstg  hgt=height
  Product : Product  RndMeth=Zero
  Product1 : Product  RndMeth=Zero
  Product2 : Product  RndMeth=Zero
  Q_in : Constant  Value=zeros(nodes,1)
  Relay : Relay  OnSwitchValue=0.05  OffSwitchValue=-0.05
  T_criteria not satisfied : Subsystem  TreatAsAtomicUnit=on
  index_to_internal_massflow : MATLABFcn  MATLABFcn=[u(2:end);0]  OutputDimensions=nodes
  massflow downwards : Subsystem  TreatAsAtomicUnit=on
  massflow upwards : Subsystem  TreatAsAtomicUnit=on
  select_Tin_2_Tout : Selector  InputPortWidth=nodes  IndexOptions=Index vector (dialog)  Indices=[idx_in_out]  OutputSizes=1
  select_Tn : Selector  InputPortWidth=nodes  IndexOptions=Index vector (dialog)  Indices=[1:nodes]  OutputSizes=1
  select_Tn_concerned : Selector  InputPortWidth=nodes  IndexOptions=Index vector (dialog)  Indices=n_concerned  OutputSizes=1
  select_Tout : Selector  InputPortWidth=nodes  IndexOptions=Index vector (dialog)  Indices=[outlet]  OutputSizes=1
  to_storeT : Outport
  THBout : Outport  Port=2
  wires:
  select_Tin_2_Tout/1 -> Pressure_Drop_StoragePipe/1
  Pressure_Drop_StoragePipe/1 -> Bus Assignment/1
  select_Tn_concerned/1 -> Add2/1, massflow downwards/1(In1), massflow upwards/1(In1)
  MinMax/1 -> Product1/2
  Add2/1 -> If/1
  Product1/1 -> Mux3/2  "mdot_in"
  Gain5/1 -> Product/2
  Relay/1 -> select_Tn_concerned/1, index_to_internal_massflow/1
  Product/1 -> Mux3/4  "mdot_down"
  from_storeT/1 -> select_Tin_2_Tout/1, select_Tn/1, select_Tout/1
  THBin/1 -> Pressure_Drop_StoragePipe/2, Bus Selector/1
  Bus Selector/4 -> Mux3/7  "<FluidType>"
  Bus Selector/3 -> Mux3/6  "<Pressure>"
  Bus Selector/2 -> Product/1, Product2/1, Product1/1  "<MassFlow>"
  Bus Selector/1 -> Gain3/1, Add/1  "<Temperature>"
  Mux3/1 -> to_storeT/1
  select_Tout/1 -> Bus Assignment/2
  Gain3/1 -> Mux3/1  "T_in"
  Q_in/1 -> Mux3/5
  Bus Assignment/1 -> THBout/1
  Bus Selector/5 -> Mux3/8  "<FluidMix>"
  select_Tn/1 -> Add/2
  Add/1 -> Gain2/1
  If/1 -> T_criteria not satisfied/Action
  Constant/1 -> If/2
  T_criteria not satisfied/1(Out1) -> MinMax/1
  If/2 -> massflow downwards/Action
  If/3 -> massflow upwards/Action
  massflow downwards/1(Out1) -> MinMax/2
  Gain1/1 -> Product2/2
  Product2/1 -> Mux3/3  "mdot_up"
  massflow upwards/1(Out1) -> MinMax/3
  Gain2/1 -> Relay/1
  index_to_internal_massflow/1 -> Gain5/1, Gain1/1

== system carnot/Storage/Thermal/Storage_Type_5/HX_EN12977_3 ==
  from_storeT : Inport
  THBin : Inport  Port=2
  Bus Assignment1 : BusAssignment  AssignedSignals=Temperature
  Mux3 : Mux  Inputs=8
  Pressure_Drop_StorageHX : $bdroot/Basic/Pressure_Drop/Pressure_Drop_StorageHX  dia=dia  hgt=height  dplin=dplin  dpqua=dpqua
  T_in : Constant  Value=zeros(nodes,1)
  fluid : Constant  Value=-9999
  mdot_in : Constant  Value=zeros(nodes,1)
  mix : Constant  Value=-9999
  p : Constant  Value=-9999
  select_Tout : Selector  InputPortWidth=nodes  IndexOptions=Index vector (dialog)  Indices=[outlet]  OutputSizes=1
  sfun_storage_heatexchanger : $bdroot/Basic/Thermal_Models/sfun_storage_heatexchanger  idn=heat transfer data fit EN12977  nodes=nodes  inlet=inlet  outlet=outlet  p1=ua0  p2=uam  p3=uat  p4=uat2  p5=0  p6=0  p7=0
  to_storeT : Outport
  THBout : Outport  Port=2
  wires:
  from_storeT/1 -> sfun_storage_heatexchanger/1
  THBin/1 -> Pressure_Drop_StorageHX/1, sfun_storage_heatexchanger/2
  mdot_in/1 -> Mux3/2, Mux3/3, Mux3/4  "mdot_in"
  Mux3/1 -> to_storeT/1
  select_Tout/1 -> Bus Assignment1/2
  T_in/1 -> Mux3/1  "T_in"
  sfun_storage_heatexchanger/1 -> Mux3/5  "Q_in"
  Bus Assignment1/1 -> THBout/1
  p/1 -> Mux3/6
  fluid/1 -> Mux3/7
  mix/1 -> Mux3/8
  sfun_storage_heatexchanger/2 -> select_Tout/1
  Pressure_Drop_StorageHX/1 -> Bus Assignment1/1

== system carnot/Storage/Thermal/detailed_storage_models/heat_exchanger_storage ==
  Tamb : Inport
  THBex_in : Inport  Port=2
  THBstg_in : Inport  Port=3
  Demux : Demux
  Demux1 : Demux  Outputs=[1 1 1 1 1 1]
  Demux2 : Demux  Outputs=[1 1 1 1 1 1]
  Demux3 : Demux  Outputs=[6 14]
  Demux4 : Demux  Outputs=[6 14]
  Mux1 : Mux  Inputs=7
  Mux2 : Mux  Inputs=7
  Mux3 : Mux  Inputs=13
  S-Function : S-Function  FunctionName=ministg  Parameters=v(1), v(2), loss, uh(1), uh(2), uc(1), uc(2), uw(1), uw(2), mat, m(1), m(2), t0, dph(1), dph(2), dph(3), dpc(1), dpc(2), dpc(3), n  SFunctionDeploymentMode=off  EnableBusSupport=off
  THB2THV : $bdroot/Toolbox/THB2THV
  THB2THV1 : $bdroot/Toolbox/THB2THV
  THV2THB : $bdroot/Toolbox/THV2THB
  THV2THB1 : $bdroot/Toolbox/THV2THB
  THBex : Outport
  THBstg : Outport  Port=2
  wires:
  Mux3/1 -> S-Function/1
  Demux2/6 -> Mux2/6, Mux3/13  "fluidmix"
  Demux1/6 -> Mux1/6, Mux3/7  "fluidmix"
  THV2THB1/1 -> THBstg/1
  THV2THB/1 -> THBex/1
  THB2THV1/1 -> Demux4/1
  THB2THV/1 -> Demux3/1
  Demux2/5 -> Mux2/5, Mux3/12  "fluidtype"
  Demux2/3 -> Mux2/3, Mux3/10  "mdot"
  Demux1/5 -> Mux1/5, Mux3/6  "fluidtype"
  Demux1/3 -> Mux1/3, Mux3/4  "mdot"
  Demux1/4 -> Mux3/5
  Demux1/2 -> Mux3/3
  Tamb/1 -> Mux3/1
  Demux1/1 -> Mux1/1, Mux3/2  "ID"
  Demux2/4 -> Mux3/11
  Demux2/2 -> Mux3/9
  Demux2/1 -> Mux2/1, Mux3/8  "ID"
  S-Function/1 -> Demux/1
  Demux3/1 -> Demux1/1
  THBex_in/1 -> THB2THV/1
  THBstg_in/1 -> THB2THV1/1
  Demux4/1 -> Demux2/1
  Demux/4 -> Mux2/4
  Demux/3 -> Mux2/2
  Mux2/1 -> THV2THB1/1
  Mux1/1 -> THV2THB/1
  Demux/2 -> Mux1/4
  Demux/1 -> Mux1/2
  Demux3/2 -> Mux1/7
  Demux4/2 -> Mux2/7

== system carnot/Storage/Thermal/surface_models/Isolated_Cover ==
  Tamb : Inport
  Mux2 : Mux  Inputs=2
  const1 : Constant  Value=[u 0]
  Tamb_utop_Iabs : Outport
  wires:
  Mux2/1 -> Tamb_utop_Iabs/1
  const1/1 -> Mux2/2
  Tamb/1 -> Mux2/1

== system carnot/Storage/Thermal/surface_models/Open_Surface ==
  WDB : Inport
  3*vwind : Gain  Gain=3  SaturateOnIntegerOverflow=on  OutDataTypeStr=Inherit: Same as input  ParamDataTypeStr=Inherit: Same as input
  Bus Selector : BusSelector  OutputSignals=Solar_Radiation_direct_surface,Solar_Radiation_diffuse_surface,Temperature_Ambient,Wind_Speed
  Fixed_Surface : $bdroot/Weather/Fixed_Surface  colangle=0  colazi=0  colrot=0
  Mux2 : Mux  Inputs=3
  Radiation_on_Inclined_Surface : $bdroot/Weather/Radiation_on_Inclined_Surface  sky=Perez 1990  reflect=0.2
  Sum : Sum  Inputs=2  SaturateOnIntegerOverflow=on  InputSameDT=on  OutDataTypeStr=Inherit: Same as first input
  add 5.6 : Subsystem  mask(add constant){c=5.6}
      mask prompts: c "constant c"
      mask help: This block adds a constant c to each element of the input vector.
      mask Help: file:///constant.htm
      mask Display: disp('+c');
  ground absorbtion : Gain  Gain=albedo  SaturateOnIntegerOverflow=on  OutDataTypeStr=Inherit: Same as input  ParamDataTypeStr=Inherit: Same as input
  Tamb_utop_Iabs : Outport
  wires:
  Bus Selector/2 -> Sum/2  "<Solar_Radiation_diffuse_surface>"
  WDB/1 -> Radiation_on_Inclined_Surface/1
  Fixed_Surface/1 -> Radiation_on_Inclined_Surface/2
  Radiation_on_Inclined_Surface/1 -> Bus Selector/1
  Bus Selector/3 -> Mux2/1  "<Temperature_Ambient>"
  ground absorbtion/1 -> Mux2/3
  Bus Selector/1 -> Sum/1  "<Solar_Radiation_direct_surface>"
  Sum/1 -> ground absorbtion/1
  3*vwind/1 -> add 5.6/1(In1)
  add 5.6/1(Out1) -> Mux2/2
  Mux2/1 -> Tamb_utop_Iabs/1
  Bus Selector/4 -> 3*vwind/1  "<Wind_Speed>"

== system carnot/Basic/Thermal_Models/Combustion_Calculation/exhaust gas/fluid//solid ==
  c : Inport
  h : Inport  Port=2
  s : Inport  Port=3
  n : Inport  Port=4
  w : Inport  Port=5
  Mux : Mux  Inputs=2
  Mux1 : Mux
  kgCO2 : Gain  Gain=3.67  SaturateOnIntegerOverflow=on  OutDataTypeStr=Inherit: Same as input  ParamDataTypeStr=Inherit: Same as input
  kgH2O : Fcn  Expr=9*u(1)+u(2)
  kgSO2 : Gain  Gain=2  SaturateOnIntegerOverflow=on  OutDataTypeStr=Inherit: Same as input  ParamDataTypeStr=Inherit: Same as input
  Out1 : Outport
  wires:
  n/1 -> Mux1/4
  s/1 -> kgSO2/1
  w/1 -> Mux/2
  Mux1/1 -> Out1/1
  h/1 -> Mux/1
  c/1 -> kgCO2/1
  kgSO2/1 -> Mux1/3
  kgH2O/1 -> Mux1/2
  kgCO2/1 -> Mux1/1
  Mux/1 -> kgH2O/1

== system carnot/Basic/Thermal_Models/Combustion_Calculation/exhaust gas/gas ==
  c : Inport
  h : Inport  Port=2
  s : Inport  Port=3
  n : Inport  Port=4
  Mux1 : Mux
  Terminator1 : Terminator
  kgCO2 : Gain  Gain=3.67  SaturateOnIntegerOverflow=on  OutDataTypeStr=Inherit: Same as input  ParamDataTypeStr=Inherit: Same as input
  kgH2O : Gain  Gain=9  SaturateOnIntegerOverflow=on  OutDataTypeStr=Inherit: Same as input  ParamDataTypeStr=Inherit: Same as input
  kgSO2 : Ground
  Out1 : Outport
  wires:
  n/1 -> Mux1/4
  kgSO2/1 -> Mux1/3
  kgH2O/1 -> Mux1/2
  kgCO2/1 -> Mux1/1
  Mux1/1 -> Out1/1
  s/1 -> Terminator1/1
  h/1 -> kgH2O/1
  c/1 -> kgCO2/1

== system carnot/Basic/Thermal_Models/HeatPump_basic/model cold side/add constant ==
  In1 : Inport
  Sum : Sum  SaturateOnIntegerOverflow=on  InputSameDT=on  OutDataTypeStr=Inherit: Same as first input
  const : Constant  Value=c
  Out1 : Outport
  wires:
  const/1 -> Sum/1
  In1/1 -> Sum/2
  Sum/1 -> Out1/1

== system carnot/Basic/Thermal_Models/Room_Node/convective_node/PressureCalculation ==
  D_mdot_air : Inport
  density : Inport  Port=2
  zoneairvolume : Inport  Port=3
  T : Inport  Port=4
  Enable : EnablePort
  Multiply : Product
  Subsystem : Subsystem
  m_air : Integrator  InitialConditionSource=external  InitialCondition=zonestartAIR  LimitOutput=on  LowerSaturationLimit=0
  x : Product  Inputs=*/*  SaturateOnIntegerOverflow=on  InputSameDT=on  OutDataTypeStr=Inherit: Same as first input
  p : Outport
  wires:
  D_mdot_air/1 -> m_air/1
  T/1 -> Subsystem/1(T)
  x/1 -> p/1
  density/1 -> Multiply/1
  m_air/1 -> x/1
  zoneairvolume/1 -> x/2, Multiply/2
  Multiply/1 -> m_air/2
  Subsystem/1(R*T ') -> x/3

== system carnot/Source/Chiller/Absorption_Chiller_LookUp/Lookup_table Q_hot + Q_cold + Recooling/NTDeadTime ==
  control_AC_runtime : Inport
  T_HT_IN : Inport  Port=2
  Compare To Constant : simulink/Logic and Bit Operations/Compare To Constant  relop=<  const=1  OutDataTypeStr=boolean
  Compare To Constant1 : simulink/Logic and Bit Operations/Compare To Constant  relop=>=  const=1  OutDataTypeStr=boolean
  Compare To Constant2 : simulink/Logic and Bit Operations/Compare To Constant  relop=>  const=eps(1)  OutDataTypeStr=boolean
  Constant : Constant  Value=data.deadtime_exponent
  Constant1 : Constant  Value=0.0
  Display{,1..3,5..6} (6 alike) : Display
  Gain_11768 : Gain  Gain=data.deadtime_factor
  Logical Operator : Logic  AllPortsSameDT=off  OutDataTypeStr=boolean
  Logical Operator1 : Logic  AllPortsSameDT=off  OutDataTypeStr=boolean
  Logical Operator2 : Logic  AllPortsSameDT=off  OutDataTypeStr=boolean
  Logical Operator3 : Logic  Operator=OR  AllPortsSameDT=off  OutDataTypeStr=boolean
  Math Function : Math  Operator=pow  SaturateOnIntegerOverflow=on
  Memory : Memory
  Memory1 : Memory
  Memory2 : Memory
  Relational Operator : RelationalOperator  OutDataTypeStr=boolean  RndMeth=Simplest
  Switch : Switch  Criteria=u2 > Threshold  Threshold=0.5
  Switch1 : Switch  Criteria=u2 > Threshold  Threshold=eps(1)
  Q_cold_on : Outport
  wires:
  T_HT_IN/1 -> Math Function/1
  Constant/1 -> Math Function/2
  Math Function/1 -> Gain_11768/1
  Gain_11768/1 -> Display/1, Switch/1
  Memory/1 -> Compare To Constant/1
  Compare To Constant/1 -> Logical Operator/1
  Logical Operator/1 -> Switch/2
  Switch/1 -> Switch1/1, Memory1/1, Display1/1
  Memory1/1 -> Switch/3
  control_AC_runtime/1 -> Display2/1, Compare To Constant2/1, Relational Operator/1, Switch1/2, Display5/1, Compare To Constant1/1, Memory/1
  Constant1/1 -> Switch1/3
  Compare To Constant1/1 -> Logical Operator/2
  Switch1/1 -> Display6/1, Relational Operator/2
  Relational Operator/1 -> Logical Operator1/2
  Compare To Constant2/1 -> Logical Operator1/1, Logical Operator2/2
  Memory2/1 -> Logical Operator2/1
  Logical Operator2/1 -> Logical Operator3/1
  Logical Operator3/1 -> Memory2/1, Display3/1, Q_cold_on/1
  Logical Operator1/1 -> Logical Operator3/2

== system carnot/Source/Chiller/Absorption_Chiller_LookUp/Lookup_table Q_hot + Q_cold + Recooling/runtime_AC ==
  control_AC : Inport
  Integrator : Integrator  ExternalReset=either
  runtime : Outport
  wires:
  control_AC/1 -> Integrator/2, Integrator/1
  Integrator/1 -> runtime/1

== system carnot/Source/Chiller/Absorption_Chiller_ddT/absorber // condenser/Tcooler_out ==
  T : Inport
  mdot : Inport  Port=2
  Qdot_E + Qdot_G : Inport  Port=3
  p : Inport  Port=4
  fluid : Inport  Port=5
  mix : Inport  Port=6
  Heat_Capacity : $bdroot/Basic/Material_Properties/Heat_Capacity  VariantControl=CarlibClassic  INPUTARGUMENTS=state variables (classic)  DEBUGLEVEL=DEBUGLEVEL  MAXTOTALWARNINGS=inf  MAXCONSECUTIVEWARNINGS=inf  WRITETOFILE=0  FILENAME='errors.txt'
  Product1 : Product  Inputs=//*  SaturateOnIntegerOverflow=on  InputSameDT=on  OutDataTypeStr=Inherit: Same as first input
  Saturation : Saturate  UpperLimit=inf  LowerLimit=1e-5
  Sum3 : Sum  SaturateOnIntegerOverflow=on  InputSameDT=on  OutDataTypeStr=Inherit: Same as first input
  Tcooler_out : Outport  InitialOutput=0
  wires:
  Qdot_E + Qdot_G/1 -> Product1/3
  Saturation/1 -> Product1/1
  Sum3/1 -> Tcooler_out/1
  mdot/1 -> Saturation/1
  Product1/1 -> Sum3/2
  Heat_Capacity/1 -> Product1/2
  T/1 -> Heat_Capacity/1, Sum3/1
  p/1 -> Heat_Capacity/2
  fluid/1 -> Heat_Capacity/3
  mix/1 -> Heat_Capacity/4

== system carnot/Source/Chiller/Absorption_Chiller_ddT/boiler/Qdot_G with deltadelta_t ==
  deltadelta_t : Inport
  Add1 : Sum
  Constant : Constant  Value=rG
  Gain1 : Gain  Gain=sG
  Transfer Fcn : TransferFcn  Denominator=[600 1]
  kW_2_W : Gain  Gain=1000
  Qdot_G [W] : Outport
  wires:
  Transfer Fcn/1 -> Qdot_G [W]/1
  kW_2_W/1 -> Transfer Fcn/1
  Add1/1 -> kW_2_W/1
  deltadelta_t/1 -> Gain1/1
  Gain1/1 -> Add1/2
  Constant/1 -> Add1/1

== system carnot/Source/Chiller/Absorption_Chiller_ddT/boiler/Thot_out ==
  Thot_in : Inport
  mdot : Inport  Port=2
  Qdot_G : Inport  Port=3
  p : Inport  Port=4
  fluid : Inport  Port=5
  mix : Inport  Port=6
  Heat_Capacity : $bdroot/Basic/Material_Properties/Heat_Capacity  VariantControl=CarlibClassic  INPUTARGUMENTS=state variables (classic)  DEBUGLEVEL=DEBUGLEVEL  MAXTOTALWARNINGS=inf  MAXCONSECUTIVEWARNINGS=inf  WRITETOFILE=0  FILENAME='errors.txt'
  Product1 : Product  Inputs=//*  SaturateOnIntegerOverflow=on  InputSameDT=on  OutDataTypeStr=Inherit: Same as first input
  Saturation : Saturate  UpperLimit=inf  LowerLimit=1e-5
  Sum3 : Sum  Inputs=+-  SaturateOnIntegerOverflow=on  InputSameDT=on  OutDataTypeStr=Inherit: Same as first input
  Thot_out : Outport  InitialOutput=0
  wires:
  Qdot_G/1 -> Product1/3
  Saturation/1 -> Product1/1
  Sum3/1 -> Thot_out/1
  mdot/1 -> Saturation/1
  Product1/1 -> Sum3/2
  Heat_Capacity/1 -> Product1/2
  Thot_in/1 -> Heat_Capacity/1, Sum3/1
  p/1 -> Heat_Capacity/2
  fluid/1 -> Heat_Capacity/3
  mix/1 -> Heat_Capacity/4

== system carnot/Source/Chiller/Absorption_Chiller_ddT/evaporator/Qdot_E with deltadelta_t ==
  deltadelta_t : Inport
  Add1 : Sum
  Constant : Constant  Value=rE
  Gain1 : Gain  Gain=sE
  Transfer Fcn : TransferFcn  Denominator=[600 1]
  kW_2_W : Gain  Gain=1000
  Qdot_E [W] : Outport
  wires:
  Transfer Fcn/1 -> Qdot_E [W]/1
  kW_2_W/1 -> Transfer Fcn/1
  Add1/1 -> kW_2_W/1
  deltadelta_t/1 -> Gain1/1
  Gain1/1 -> Add1/2
  Constant/1 -> Add1/1

== system carnot/Source/Chiller/Absorption_Chiller_ddT/evaporator/Tchilled_out ==
  note: Qdot_chilled_out = Qdot_chilled_in - Q_E
      | tchilled_out = Tchilled_in * mdot* cp - Qdot_E / (mdot * cp)
  T : Inport
  mdot : Inport  Port=2
  Qdot_E : Inport  Port=3
  p : Inport  Port=4
  fluid : Inport  Port=5
  mix : Inport  Port=6
  Heat_Capacity : $bdroot/Basic/Material_Properties/Heat_Capacity  VariantControl=CarlibClassic  INPUTARGUMENTS=state variables (classic)  DEBUGLEVEL=DEBUGLEVEL  MAXTOTALWARNINGS=inf  MAXCONSECUTIVEWARNINGS=inf  WRITETOFILE=0  FILENAME='errors.txt'
  Product1 : Product  Inputs=//*  SaturateOnIntegerOverflow=on  InputSameDT=on  OutDataTypeStr=Inherit: Same as first input
  Saturation : Saturate  UpperLimit=inf  LowerLimit=1e-5
  Sum3 : Sum  Inputs=+-  SaturateOnIntegerOverflow=on  InputSameDT=on  OutDataTypeStr=Inherit: Same as first input
  Tcold : Outport  InitialOutput=0
  wires:
  Product1/1 -> Sum3/2
  Qdot_E/1 -> Product1/3
  mdot/1 -> Saturation/1
  Saturation/1 -> Product1/1
  Sum3/1 -> Tcold/1
  Heat_Capacity/1 -> Product1/2
  T/1 -> Heat_Capacity/1, Sum3/1
  p/1 -> Heat_Capacity/2
  fluid/1 -> Heat_Capacity/3
  mix/1 -> Heat_Capacity/4

== system carnot/Source/Chiller/Compression_Air_Water_Chiller/Lookup_tables _COP + Q_cold_faktor/runtime_AC ==
  control_AC : Inport
  Integrator : Integrator  ExternalReset=either  InitialCondition=1
  runtime : Outport
  wires:
  control_AC/1 -> Integrator/2, Integrator/1
  Integrator/1 -> runtime/1

== system carnot/Source/Chiller/Cooling_Tower/Feuchtkugel- temperatureinfluss // wet-bulb temperature effect/Abgleich  ==
  note: Durch den Abgleich der vorliegenden Datensätze
      | wierd die Annahme getroffen
      | das bei einer reduzierung der Feuchtkugeltemp um 1K
      |  sich die Kaltwassertemp um 0.27K sinkt.
      |
      | y = ((t_FK-15)*0.27)+t_ia_100
      |
      | Ab eine Eintritstemperatur von 41 °C wierd mit
      | dem Faktor 0,25 K gerechnet.
      |
      | y = ((t_FK-15)*0.25)+t_ia_100
  t_FK : Inport
  t_ie : Inport  Port=2
  t_ia_FK15 : Inport  Port=3
  Embedded MATLAB Function : MATLAB Function  TreatAsAtomicUnit=on
  t_ia_FK : Outport
  wires:
  Embedded MATLAB Function/1(y) -> t_ia_FK/1
  t_FK/1 -> Embedded MATLAB Function/1(t_fk)
  t_ia_FK15/1 -> Embedded MATLAB Function/2(t_ia_fk15)
  t_ie/1 -> Embedded MATLAB Function/3(t_ie)

== system carnot/Source/Chiller/Cooling_Tower/Feuchtkugel- temperatureinfluss // wet-bulb temperature effect/wet-bulb 15 °C ==
  t_ie : Inport
  Lookup Table : Lookup  InputValues=[26 28 30 32 34 36 38 40 42 44 79.2]  Table=[22.6 23.9 25.2 26.4 27.7 28.9 30.1 31.2 32.4 33.5 49.25]
  t_ia_FK15 : Outport
  wires:
  t_ie/1 -> Lookup Table/1
  Lookup Table/1 -> t_ia_FK15/1

== system carnot/Source/Chiller/Cooling_Tower/Leistungseinflüsse // influence on coolingpower/Qdot_i_FK ==
  t_ia_FK : Inport
  t_ie : Inport  Port=2
  Fluid_Type : Inport  Port=3
  Add : Sum
  Constant : Constant  Value=0.3
  Constant1 : Constant  Value=2.4
  Constant2 : Constant  Value=2
  Density : $bdroot/Basic/Material_Properties/Density  VariantControl=CarlibClassic  INPUTARGUMENTS=state variables (classic)  DEBUGLEVEL=DEBUGLEVEL  MAXTOTALWARNINGS=inf  MAXCONSECUTIVEWARNINGS=inf  WRITETOFILE=0  FILENAME='errors.txt'
  Divide1 : Product  Inputs=*/
  Divide2 : Product  Inputs=*/
  Divide3 : Product  Inputs=*/
  Heat_Capacity : $bdroot/Basic/Material_Properties/Heat_Capacity  VariantControl=CarlibClassic  INPUTARGUMENTS=state variables (classic)  DEBUGLEVEL=DEBUGLEVEL  MAXTOTALWARNINGS=inf  MAXCONSECUTIVEWARNINGS=inf  WRITETOFILE=0  FILENAME='errors.txt'
  Product : Product  Inputs=4  RndMeth=Zero
  Subtract : Sum  Inputs=+-
  phi_Le1 : Constant  Value=1000
  phi_Le2 : Constant  Value=1000
  phi_Le3 : Constant  Value=1e5
  Qdot_i_FK : Outport
  wires:
  t_ia_FK/1 -> Subtract/2, Add/2
  Product/1 -> Qdot_i_FK/1
  Subtract/1 -> Product/1
  t_ie/1 -> Density/1, Subtract/1, Add/1
  Constant/1 -> Heat_Capacity/4, Density/4
  Density/1 -> Divide2/1
  phi_Le3/1 -> Heat_Capacity/2, Density/2
  Fluid_Type/1 -> Heat_Capacity/3, Density/3
  phi_Le1/1 -> Divide2/2
  Divide2/1 -> Product/4
  Constant1/1 -> Product/3
  Heat_Capacity/1 -> Divide3/1
  Constant2/1 -> Divide1/2
  Divide1/1 -> Heat_Capacity/1
  Add/1 -> Divide1/1
  phi_Le2/1 -> Divide3/2
  Divide3/1 -> Product/2

== system carnot/Source/Chiller/Cooling_Tower/Leistungseinflüsse // influence on coolingpower/Qdot_i_ist  ==
  Qdot_i_FK : Inport
  n_Fan [%] : Inport  Port=2
  Fluid_mix : Inport  Port=3
  mdot_i : Inport  Port=4
  Fluid_Type : Inport  Port=5
  t_ie : Inport  Port=6
  Constant : Constant  Value=92
  Constant2 : Constant  Value=100
  Density : $bdroot/Basic/Material_Properties/Density  VariantControl=CarlibClassic  INPUTARGUMENTS=state variables (classic)  DEBUGLEVEL=DEBUGLEVEL  MAXTOTALWARNINGS=inf  MAXCONSECUTIVEWARNINGS=inf  WRITETOFILE=0  FILENAME='errors.txt'
  Divide : Product  Inputs=**/
  Divide1 : Product  Inputs=*/
  Divide2 : Product  Inputs=*/
  Lookup Table (2-D) Volumenstromänderung : Lookup2D  RowIndex=[1.07 1.77 2.4 2.65 3.03]  ColumnIndex=[25 30 35 40 45 50 55 60 65]  Table=[0.7248 0.7054 0.6860 0.6666 0.6472 0.6278 0.6084 0.5890 0.5696; 0.9493 0.9294 0.9096 0.8897 0.8698 0.8500 0.8301 0.8103 0.7904; 1 1 1 1 1 1 1 1 1; 1.1191 1.1295 1.0956 1.0674 1.0450 1.0284 1.0175 1.0123 1.0129; 1.2370 1.1910 1.1526 1.1219 1.0988 1.0833 1.0754 1.0752 1.0826]
  Lookup Table Lüfterdrehzahl : Lookup  InputValues=[0 0.2 0.3 0.5 0.7 0.9 1]  Table=[0 0.37 0.482 0.625 0.786 0.928 1]
  Lookup Table1 Glykol : Lookup  InputValues=[0 0.1 0.2 0.3 0.4 0.5 0.6 0.7 0.8 0.9 1]  Table=[1 0.98 0.95 0.92 0.875 0.83 0.78 0.73 0.68 0.63 0.57]
  Product : Product  RndMeth=Zero
  Product1 : Product  RndMeth=Zero
  Product2 : Product  RndMeth=Zero
  phi_Le1 : Constant  Value=1000
  phi_Le3 : Constant  Value=1e5
  Qdot_i_ist : Outport
  wires:
  n_Fan [%]/1 -> Lookup Table Lüfterdrehzahl/1
  Lookup Table Lüfterdrehzahl/1 -> Product/2
  Qdot_i_FK/1 -> Product/1
  Product/1 -> Divide/1
  Product1/1 -> Product2/1
  Lookup Table1 Glykol/1 -> Product2/2
  Fluid_mix/1 -> Density/4, Lookup Table1 Glykol/1
  Divide/1 -> Product1/1
  Constant/1 -> Divide/3
  mdot_i/1 -> Divide1/1
  Product2/1 -> Qdot_i_ist/1
  Density/1 -> Divide2/1
  phi_Le3/1 -> Density/2
  Fluid_Type/1 -> Density/3
  phi_Le1/1 -> Divide2/2
  Divide2/1 -> Divide1/2
  t_ie/1 -> Density/1, Lookup Table (2-D) Volumenstromänderung/2  "column"
  Divide1/1 -> Lookup Table (2-D) Volumenstromänderung/1  "row"
  Lookup Table (2-D) Volumenstromänderung/1 -> Product1/2
  Constant2/1 -> Divide/2
